simulink model "my_gm_HDLModulatorFull"  (R2024a)
settings: Solver=FixedStepDiscrete  StartTime=0.0  StopTime=stopTime  RelTol=1e-3
values from neighbouring files (symbols this model uses):
  dataSymbols = [ ... (first row only)    [testModulatorFull.m]
undefined symbols (not defined in the file or in its folder): fPHY, fs, interpolatorFilter, numDataCarriers
libraries: dspsigops x56, hdlmdlgenlib x56, hdlsllib x8, dspsrcs4 x4, commdigbbndam3 x2, whdlutilities x1, commdigbbndpm3 x1, dsphdlsigops2 x1, dsphdlfiltering2 x1, whdlmod x1, HDL_ieee_8021513 x1
(part 2 of 2)

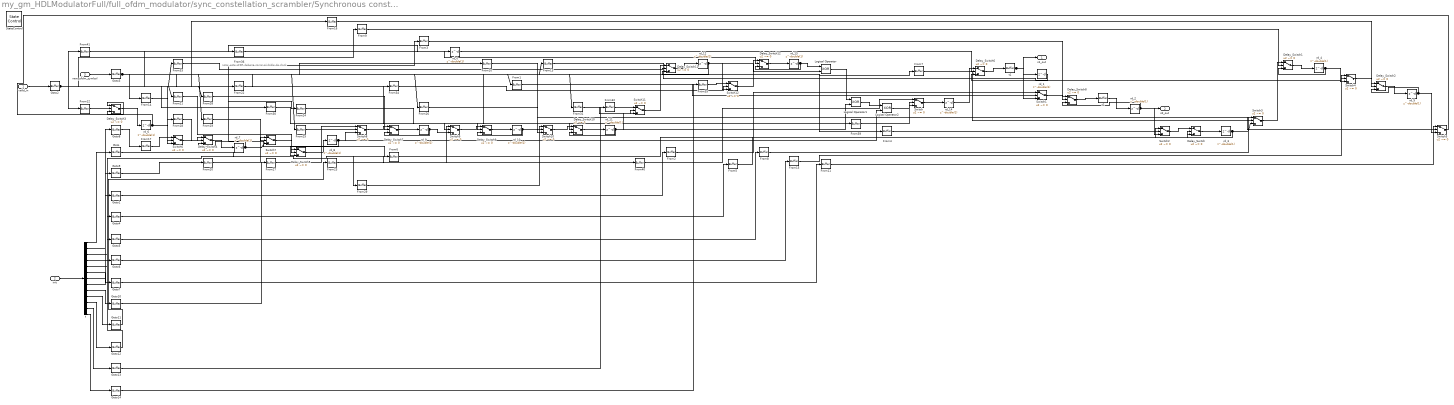
== system my_gm_HDLModulatorFull/full_ofdm_modulator/sync_constellation_scrambler/Synchronous constellation scrambler ==
  note: nota: este LFSR deberia correr al doble de clock
  valid_in : Inport  OutDataTypeStr=boolean  PortDimensions=1  SampleTime=1e-08
  init : Inport  Port=2  OutDataTypeStr=boolean  PortDimensions=[1 13]  SampleTime=1e-08
  new_ofdm_symbol : Inport  Port=3  OutDataTypeStr=boolean  PortDimensions=1  SampleTime=1e-08
  Delay_Switch{,1..12} (13 alike) : Switch  Criteria=u2 ~= 0  Threshold=double(0)  OutDataTypeStr=boolean  SampleTime=1e-08  SaturateOnIntegerOverflow=off  InputSameDT=off
  From{1..36,39..41} (39 alike) : hdlmdlgenlib/Buffer
  Goto{,1..14} (15 alike) : hdlmdlgenlib/Buffer
  Logical Operator : Logic  Operator=XOR  AllPortsSameDT=off  OutDataTypeStr=boolean  SampleTime=1e-08
  Logical Operator1 : Logic  Operator=XOR  AllPortsSameDT=off  OutDataTypeStr=boolean  SampleTime=1e-08
  Logical Operator2 : Logic  Operator=XOR  AllPortsSameDT=off  OutDataTypeStr=boolean  SampleTime=1e-08
  StateControl : StateControl  StateControl=Synchronous
  Switch{,1..12} (13 alike) : Switch  Criteria=u2 ~= 0  Threshold=double(0)  OutDataTypeStr=boolean  SampleTime=1e-08  SaturateOnIntegerOverflow=off  InputSameDT=off
  rd_{0..14} (15 alike) : Delay  DelayLength=double(1)  InitialCondition=0  SampleTime=1e-08
  t : Demux  Outputs=13
  t1 : hdlmdlgenlib/Buffer
  t2 : hdlmdlgenlib/Buffer
  s1_out : Outport  SampleTime=1e-08  VectorParamsAs1DForOutWhenUnconnected=off
  s2_out : Outport  Port=2  SampleTime=1e-08  VectorParamsAs1DForOutWhenUnconnected=off
  wires:
  valid_in/1 -> Goto2/1
  init/1 -> t/1
  new_ofdm_symbol/1 -> Goto3/1
  t1/1 -> rd_1/1, s1_out/1, Switch1/3
  Goto3/1 -> From7/1, From4/1, From39/1, From34/1, From31/1, From26/1, From25/1, From22/1, From19/1, From14/1, From13/1, From10/1, From1/1
  Goto7/1 -> From11/1
  Goto2/1 -> From9/1, From6/1, From41/1, From36/1, From33/1, From30/1, From3/1, From28/1, From24/1, From21/1, From18/1, From16/1, From12/1
  Goto6/1 -> From15/1
  Goto8/1 -> From17/1
  Goto1/1 -> From2/1
  Goto9/1 -> From20/1
  Goto11/1 -> From23/1
  Goto10/1 -> From27/1
  Goto12/1 -> From29/1
  Goto13/1 -> From32/1
  Goto14/1 -> From35/1
  Goto/1 -> From40/1
  Goto4/1 -> From5/1
  Goto5/1 -> From8/1
  t/1 -> Goto/1
  t/2 -> Goto1/1
  t/3 -> Goto4/1
  t/4 -> Goto5/1
  t/5 -> Goto6/1
  t/6 -> Goto7/1
  t/7 -> Goto8/1
  t/8 -> Goto9/1
  t/9 -> Goto10/1
  t/10 -> Goto11/1
  t/11 -> Goto12/1
  t/12 -> Goto13/1
  t/13 -> Goto14/1
  From5/1 -> Switch2/1
  From4/1 -> Switch2/2
  From6/1 -> Delay_Switch/2
  From8/1 -> Switch3/1
  From7/1 -> Switch3/2
  From9/1 -> Delay_Switch1/2
  From15/1 -> Switch4/1
  From13/1 -> Switch4/2
  From16/1 -> Delay_Switch2/2
  From11/1 -> Switch5/1
  From10/1 -> Switch5/2
  From12/1 -> Delay_Switch3/2
  From17/1 -> Switch6/1
  From14/1 -> Switch6/2
  From18/1 -> Delay_Switch4/2
  From20/1 -> Switch7/1
  From19/1 -> Switch7/2
  From21/1 -> Delay_Switch5/2
  From40/1 -> Switch/1
  From39/1 -> Switch/2
  From41/1 -> rd_0/1
  From27/1 -> Switch8/1
  From25/1 -> Switch8/2
  From28/1 -> Delay_Switch7/2
  From2/1 -> Switch1/1
  From1/1 -> Switch1/2
  From3/1 -> Delay_Switch8/2
  From23/1 -> Switch9/1
  From22/1 -> Switch9/2
  From24/1 -> Delay_Switch9/2
  From29/1 -> Switch10/1
  From26/1 -> Switch10/2
  From30/1 -> Delay_Switch10/2
  From32/1 -> Switch11/1
  From31/1 -> Switch11/2
  From33/1 -> Delay_Switch11/2
  From35/1 -> Switch12/1
  From34/1 -> Switch12/2
  From36/1 -> Delay_Switch12/2
  Switch2/1 -> Delay_Switch/1
  Switch3/1 -> Delay_Switch1/1
  Switch4/1 -> Delay_Switch2/1
  Switch5/1 -> Delay_Switch3/1
  Switch6/1 -> Delay_Switch4/1
  Switch7/1 -> Delay_Switch5/1
  Switch8/1 -> Delay_Switch7/1
  Switch9/1 -> Delay_Switch9/1
  Switch10/1 -> Delay_Switch10/1
  Switch11/1 -> Delay_Switch11/1
  Switch12/1 -> Delay_Switch12/1
  Delay_Switch6/1 -> t1/1
  Logical Operator/1 -> Logical Operator1/1
  Logical Operator1/1 -> Logical Operator2/1
  Logical Operator2/1 -> Switch/3
  Switch/1 -> rd_14/1
  Delay_Switch8/1 -> t2/1
  Switch1/1 -> Delay_Switch8/1
  rd_0/1 -> Delay_Switch6/2
  rd_14/1 -> Delay_Switch6/1
  rd_1/1 -> Delay_Switch6/3
  t2/1 -> rd_2/1
  rd_2/1 -> Switch2/3, s2_out/1, Delay_Switch8/3
  Delay_Switch/1 -> rd_3/1
  rd_3/1 -> Switch3/3, Delay_Switch/3
  Delay_Switch1/1 -> rd_4/1
  rd_4/1 -> Switch4/3, Delay_Switch1/3
  Delay_Switch2/1 -> rd_5/1
  rd_5/1 -> Switch5/3, Delay_Switch2/3
  Delay_Switch3/1 -> rd_6/1
  rd_6/1 -> Switch6/3, Delay_Switch3/3
  Delay_Switch4/1 -> rd_7/1
  rd_7/1 -> Switch7/3, Delay_Switch4/3
  Delay_Switch5/1 -> rd_8/1
  rd_8/1 -> Logical Operator2/2, Switch8/3, Delay_Switch5/3
  Delay_Switch7/1 -> rd_9/1
  rd_9/1 -> Delay_Switch7/3, Switch9/3
  Delay_Switch9/1 -> rd_10/1
  rd_10/1 -> Switch10/3, Delay_Switch9/3
  Delay_Switch10/1 -> rd_11/1
  rd_11/1 -> Logical Operator1/2, Switch11/3, Delay_Switch10/3
  Delay_Switch11/1 -> rd_12/1
  rd_12/1 -> Switch12/3, Delay_Switch11/3, Logical Operator/2
  Delay_Switch12/1 -> rd_13/1
  rd_13/1 -> Delay_Switch12/3, Logical Operator/1

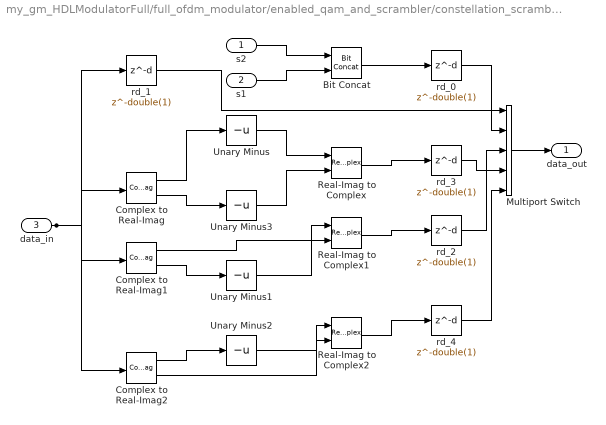
== system my_gm_HDLModulatorFull/full_ofdm_modulator/enabled_qam_and_scrambler/constellation_scrambler/rotate ==
  s2 : Inport  OutDataTypeStr=boolean  PortDimensions=1  SampleTime=1e-08
  s1 : Inport  Port=2  OutDataTypeStr=boolean  PortDimensions=1  SampleTime=1e-08
  data_in : Inport  Port=3  OutDataTypeStr=fixdt(1, 16, 14)  PortDimensions=1  SampleTime=1e-08
      settings: SignalType=complex
  Bit Concat : hdlsllib/Logic and Bit Operations/Bit Concat  numInputs=2
  Complex to Real-Imag : ComplexToRealImag  SampleTime=1e-08
  Complex to Real-Imag1 : ComplexToRealImag  SampleTime=1e-08
  Complex to Real-Imag2 : ComplexToRealImag  SampleTime=1e-08
  Multiport Switch : MultiPortSwitch  DataPortOrder=Zero-based contiguous  Inputs=4  DiagnosticForDefault=None  zeroidx=on  OutDataTypeStr=fixdt(1, 16, 14)  SampleTime=1e-08  SaturateOnIntegerOverflow=off  InputSameDT=off
  Real-Imag to Complex : RealImagToComplex  ConstantPart="fi(0,1,16,14,\"hex\",\"0000\")"  SampleTime=1e-08
  Real-Imag to Complex1 : RealImagToComplex  ConstantPart="fi(0,1,16,14,\"hex\",\"0000\")"  SampleTime=1e-08
  Real-Imag to Complex2 : RealImagToComplex  ConstantPart="fi(0,1,16,14,\"hex\",\"0000\")"  SampleTime=1e-08
  Unary Minus{,1..3} (4 alike) : UnaryMinus  SampleTime=1e-08
  rd_{0..4} (5 alike) : Delay  DelayLength=double(1)  InitialCondition=0
  data_out : Outport  SampleTime=1e-08  InitialOutput=0
  wires:
  s2/1 -> Bit Concat/1
  s1/1 -> Bit Concat/2
  data_in/1 -> rd_1/1, Complex to Real-Imag2/1, Complex to Real-Imag1/1, Complex to Real-Imag/1
  Bit Concat/1 -> rd_0/1
  Complex to Real-Imag/1 -> Unary Minus/1
  Complex to Real-Imag/2 -> Unary Minus3/1
  Complex to Real-Imag1/1 -> Real-Imag to Complex1/2
  Complex to Real-Imag1/2 -> Unary Minus1/1
  Complex to Real-Imag2/1 -> Unary Minus2/1
  Complex to Real-Imag2/2 -> Real-Imag to Complex2/1
  Multiport Switch/1 -> data_out/1
  Real-Imag to Complex/1 -> rd_3/1
  Real-Imag to Complex1/1 -> rd_2/1
  Real-Imag to Complex2/1 -> rd_4/1
  Unary Minus/1 -> Real-Imag to Complex/1
  Unary Minus1/1 -> Real-Imag to Complex1/1
  Unary Minus2/1 -> Real-Imag to Complex2/2
  Unary Minus3/1 -> Real-Imag to Complex/2
  rd_1/1 -> Multiport Switch/2
  rd_0/1 -> Multiport Switch/1
  rd_3/1 -> Multiport Switch/4
  rd_2/1 -> Multiport Switch/3
  rd_4/1 -> Multiport Switch/5

== system my_gm_HDLModulatorFull/full_ofdm_modulator/enabled_qam_and_scrambler/qam_mod/BPSK Modulator Baseband ==
  in0 : Inport  OutDataTypeStr=fixdt(0, 1, 0)  SampleTime=2e-08
  Enable_out9 : EnablePort  OutDataTypeStr=boolean
  BPSK Modulator Baseband : commdigbbndpm3/BPSK Modulator Baseband  Ph=0  outDtype=Fixed-point  outWordLen=16  outUDDataType=sfix(16)  outFracLenMode=User-defined  outFracLen=14  outDataTypeStr=fixdt(1,16,14)  outLastDataTypeStr=fixdt(1,16,14)
      settings: LibrarySourceBlock=|
      | commhdldigbbndpm/BPSK
      | Modulator
      | Baseband
  out0 : Outport  OutDataTypeStr=fixdt(1, 16, 14)  SampleTime=2e-08  InitialOutput=0
      settings: SignalType=complex
  wires:
  BPSK Modulator Baseband/1 -> out0/1
  in0/1 -> BPSK Modulator Baseband/1

== system my_gm_HDLModulatorFull/full_ofdm_modulator/enabled_qam_and_scrambler/qam_mod/batID 1 ==
  in0 : Inport  OutDataTypeStr=fixdt(0, 2, 0)  SampleTime=2e-08
  Enable_out9 : EnablePort  OutDataTypeStr=boolean
  batID 1 : commdigbbndam3/Rectangular QAM Modulator Baseband  M=4  InType=Integer  Enc=User-defined  Mapping=qamTwoBits  PowType=Average Power  MinDist=2  AvgPow=1  PeakPow=1  Ph=0  outDtype=Fixed-point  outWordLen=16  outUDDataType=sfix(16)  outFracLenMode=User-defined  outFracLen=14  outDataTypeStr=fixdt(1,16,14)  outLastDataTypeStr=fixdt(1,16,14)
      settings: LibrarySourceBlock=|
      | commhdldigbbndam/Rectangular QAM
      | Modulator
      | Baseband
  out0 : Outport  OutDataTypeStr=fixdt(1, 16, 14)  SampleTime=2e-08  InitialOutput=0
      settings: SignalType=complex
  wires:
  batID 1/1 -> out0/1
  in0/1 -> batID 1/1

== system my_gm_HDLModulatorFull/full_ofdm_modulator/enabled_qam_and_scrambler/qam_mod/batID 8 ==
  in0 : Inport  OutDataTypeStr=fixdt(0, 4, 0)  SampleTime=2e-08
  Enable_out9 : EnablePort  OutDataTypeStr=boolean
  batID 8 : commdigbbndam3/Rectangular QAM Modulator Baseband  M=16  InType=Integer  Enc=User-defined  Mapping=qamFourBits  PowType=Average Power  MinDist=2  AvgPow=1  PeakPow=1  Ph=0  outDtype=Fixed-point  outWordLen=16  outUDDataType=sfix(16)  outFracLenMode=User-defined  outFracLen=14  outDataTypeStr=fixdt(1,16,14)  outLastDataTypeStr=fixdt(1,16,14)
      settings: LibrarySourceBlock=|
      | commhdldigbbndam/Rectangular QAM
      | Modulator
      | Baseband
  out0 : Outport  OutDataTypeStr=fixdt(1, 16, 14)  SampleTime=2e-08  InitialOutput=0
      settings: SignalType=complex
  wires:
  batID 8/1 -> out0/1
  in0/1 -> batID 8/1
